simulink model "DrivetrainHevP2"  (R2018a)
settings: Solver=VariableStepAuto  StartTime=0.0  StopTime=inf  RelTol=1e-3  EnableMultiTasking=on
model workspace (MAT data in the model file):
  Aeff = 0.0314159265359
  Af = 2.46
  Bx = 10
  Cd = 0.25
  Cl = 0.1
  Cpm = 0.1
  Cx = 1.65
  Dx = 1
  Ex = 0.01
  FZMAX = 6570
  FZMIN = 0
  Fc = 500
  FsbF = [-700000 -7000 -700 0 700 7000 700000]
  FsbR = [-700000 -7000 -700 0 700 7000 700000]
  FskF = [-8928.57142857 -178.571428571 0 357.142857143 535.714285714 9285.71428571]
  FskR = [-5357.14285714 -107.142857143 0 214.285714286 321.428571429 5571.42857143]
  G = [0 1 2 3 4 5 6]
  G_o = 1
  Iyy = 3000
  Iyy_Whl = 0.8
  J = 0.01
  Jd = 0.025
  Jin = 0.05
  Jin_Cltch = 0.2
  Jin_Cltch2 = 0.01
  Jout = [0.01 0.01 0.01 0.01 0.01 0.01 0.01]
  Jout_Cltch = 0.01
  Jout_Cltch2 = 0.05
  Jw1 = 0.01
  Jw2 = 0.01
  K_c = 10000
  Lrel = 0.15
  Mass = 1623
  N = [1 4.212 2.637 1.8 1.386 1 0.772]
  NF = 2
  NR = 2
  Ndiff = 3.32
  Ndisk = 1
  Ndisks = 4
  Pabs = 101325
  Press = 7000000
  Re = 0.327
  Reff = 0.11
  Reff_LSD = 0.2
  Rm = 0.15
  T = 273
  UNLOADED_RADIUS = 0.336
  VXLOW = 2
  aMy = 0.01
  a_CG = 1.09
  alphaMy = 0
  b = Simulink.Parameter
  b.Value = 100
  b.DataType = 'auto'
  b.Dimensions = [1 1]
  b1 = 100
  b2 = 100
  bMy = 0
  b_CG = 1.7
  b_J = 0.001
  bd = 0.001
  betaMy = 1
  bin = 0.003
  bin_Cltch = 0.003
  bout = [0.003 0.003 0.003 0.003 0.003 0.003 0.003]
  bout_Cltch = 0.003
  br = 0.001
  bw1 = 0.001
  bw2 = 0.001
  cMy = 0
  disk_abore = 0.05
  domega_o = 0
  dw = [0 10 20 40 60 80 100]
  dzdotsF = [-10 -1 -0.1 0 0.1 1 10]
  dzdotsR = [-10 -1 -0.1 0 0.1 1 10]
  dzsF = [-0.005 -0.0001 0 0.2 0.2001 0.2051]
  dzsR = [-0.005 -0.0001 0 0.2 0.2001 0.2051]
  eta = [0.95 0.95 0.95 0.95 0.95 0.95 0.95]
  g = 9.81
  h = 0.5
  k = Simulink.Parameter
  k.Value = 5000
  k.DataType = 'auto'
  k.Dimensions = [1 1]
  k1 = 50000
  k2 = 50000
  kappamax = 1.5
  lam_x = 1
  mu_kinetic = 0.35
  mu_static = 0.45
  muc = [0.16 0.13 0.115 0.11 0.105 0.1025 0.10125]
  muk = 0.4
  mus = 0.45
  num_pads = 2
  omega1_c = 3000
  omega2_c = 3000
  omega_c = Simulink.Parameter
  omega_c.Value = 100
  omega_c.DataType = 'auto'
  omega_c.Dimensions = [1 1]
  omega_o_J = 0
  omegain_o = 0
  omegao = 0
  omegaout_o = 0
  omegaw1o = 0
  omegaw2o = 0
  press = 234400
  q_o = 0
  tauC = 0.1
  tauC_1 = 0.01
  tauC_LSD = 0.01
  tau_s = 0.1
  tc = 0.01
  theta_o = 0
  theta_o_Veh = 0
  ts = 0.01
  win_o = 0
  wout_o = 0
  x_o = 0
  xdot_o = 0
  z_o = -0.35
  zdot_o = 0
libraries: autolibsharedcoupling x8, autolibshared x7, autolibshareddiff x4, autolibtransamt x1, autolibcoupling x1
(part 1 of 4)
settings Model: ModifiedByFormat=The MathWorks, Inc.  PauseTimes=10  Creator=The MathWorks, Inc.  LastModifiedBy=The MathWorks, Inc.
settings SolverCC: AutoInsertRateTranBlk=on  DecoupledContinuousIntegration=on
settings DataIOCC: DSMLogging=off
settings ModelReferenceCC: PropagateSignalLabelsOutOfModel=off
settings CodeAppCC: StateflowObjectComments=on
settings GRTTargetCC: TargetLangStandard=C89/C90 (ANSI)
settings ConfigComp: CovMetricSettings=dsw  CovHtmlReporting=on  CovSaveCumulativeToWorkspaceVar=on  CovSaveSingleToWorkspaceVar=on  CovShowResultsExplorer=off  CovExternalEMLEnable=off
settings SimscapeCC: SimscapeNormalizeSystem=off

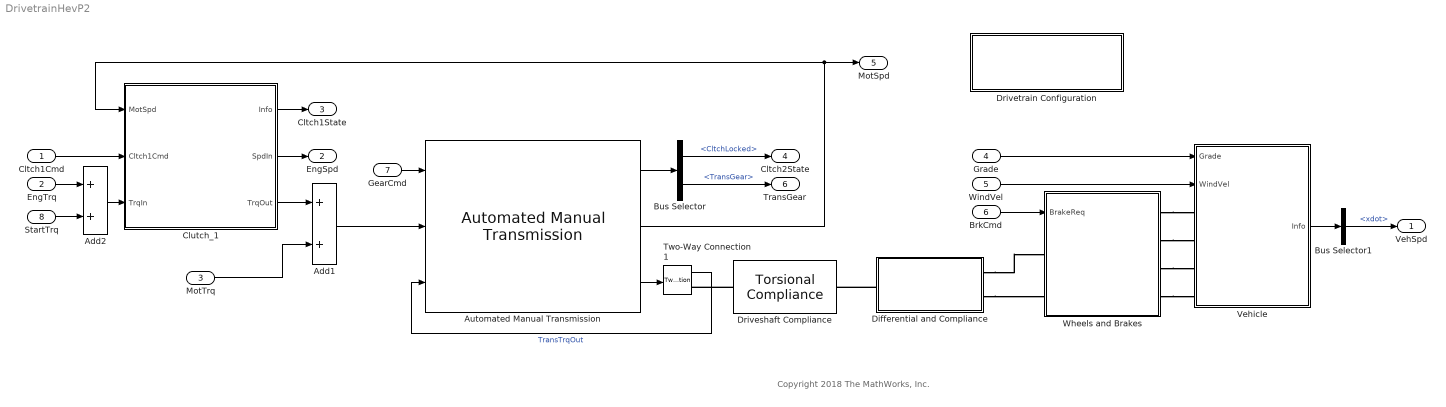
== system DrivetrainHevP2 ==
  note: Copyright 2018 The MathWorks, Inc.
  Cltch1Cmd : Inport
  EngTrq : Inport  Port=2
  MotTrq : Inport  Port=3
  Grade : Inport  Port=4
  WindVel : Inport  Port=5
  BrkCmd : Inport  Port=6
  GearCmd : Inport  Port=7
  StartTrq : Inport  Port=8
  Add1 : Sum
  Add2 : Sum
  Automated Manual Transmission : autolibtransamt/Automated Manual Transmission  VariantControl=0  cntrlType=Ideal integrated controller  TransEffModelPopup=Gear only  Jin=Jin  bin=bin  omegain_o=omegain_o  G=G  Trq_bpts=[25, 50, 75, 100, 150, 200, 250]  omega_bpts=[52.4 78.5 105 131 157 183 209 262 314 419 524]  Temp_bpts=[313 358]  N=N  Jout=Jout  bout=bout  eta=eta  eta_tbl=reshape([0.53 0.71 0.77 0.79 0.82 0.82 0.82 0.5 0.7 0.77 0.79 0.82 0.82 0.82 0.54 0.72 0.78 0.81 0.83 0.82 0.82 0.56 0.73 0.79 0.81 0.84 0.82 0.82 0.58 0.74 0.79 0.82 0.84 0.82 0.82 0.57 0.74 0.79 0.82 0.84 0.82 0.82 0.58 0.74 0.79 0.82 0.84 0.82 0.82 0.58 0.74 0.79 0.82 0.84 0.82 0.82 0.57 0.74 0.8 0.82 0.85 0.82 0.82 0.55 0.73 0.78 0.81 0.84 0.82 0.82 0.51 0.71 0.77 0.81 0.84 0.82 0.82 0.53 0.71 0.77 0.79 0.82 0.82 0.82 0.5 0.7 0.77 0.79 0.82 0.82 0.82 0.54 0.72 0.78 0.81 0.83 0.82 0.82 0.56 0.73 0.79 0.81 0.84 0.82 0.82 0.58 0.74 0.79 0.82 0.84 0.82 0.82 0.57 0.74 0.79 0.82 0.84 0.82 0.82 0.58 0.74 0.79 0.82 0.84 0.82 0.82 0.58 0.74 0.79 0.82 0.84 0.82 0.82 0.57 0.74 0.8 0.82 0.85 0.82 0.82 0.55 0.73 0.78 0.81 0.84 0.82 0.82 0.51 0.71 0.77 0.81 0.84 0.82 0.82 0.53 0.71 0.77 0.79 0.82 0.82 0.82 0.5 0.7 0.77 0.79 0.82 0.82 0.82 0.54 0.72 0.78 0.81 0.83 0.82 0.82 0.56 0.73 0.79 0.81 0.84 0.82 0.82 0.58 0.74 0.79 0.82 0.84 0.82 0.82 0.57 0.74 0.79 0.82 0.84 0.82 0.82 0.58 0.74 0.79 0.82 0.84 0.82 0.82 0.58 0.74 0.79 0.82 0.84 0.82 0.82 0.57 0.74 0.8 0.82 0.85 0.82 0.82 0.55 0.73 0.78 0.81 0.84 0.82 0.82 0.51 0.71 0.77 0.81 0.84 0.82 0.82 0.7 0.79 0.82 0.83 0.84 0.84 0.84 0.63 0.76 0.8 0.82 0.83 0.84 0.84 0.58 0.74 0.79 0.81 0.83 0.84 0.84 0.58 0.74 0.79 0.81 0.83 0.84 0.84 0.58 0.74 0.79 0.81 0.84 0.84 0.84 0.57 0.73 0.78 0.81 0.84 0.85 0.84 0.57 0.73 0.79 0.81 0.84 0.85 0.84 0.56 0.73 0.78 0.81 0.83 0.85 0.84 0.55 0.73 0.78 0.81 0.84 0.85 0.84 0.52 0.71 0.77 0.8 0.83 0.85 0.84 0.48 0.69 0.76 0.79 0.83 0.84 0.84 0.64 0.76 0.8 0.81 0.83 0.84 0.84 0.56 0.73 0.78 0.8 0.83 0.84 0.84 0.54 0.71 0.77 0.8 0.82 0.84 0.84 0.53 0.71 0.77 0.8 0.83 0.84 0.84 0.51 0.71 0.77 0.8 0.83 0.84 0.85 0.52 0.7 0.77 0.8 0.83 0.84 0.85 0.51 0.71 0.76 0.79 0.83 0.84 0.85 0.5 0.69 0.76 0.79 0.82 0.84 0.85 0.45 0.68 0.75 0.78 0.82 0.84 0.85 0.43 0.67 0.74 0.78 0.81 0.83 0.84 0.38 0.63 0.71 0.75 0.8 0.82 0.83 0.65 0.79 0.84 0.85 0.88 0.89 0.89 0.56 0.75 0.81 0.83 0.86 0.88 0.89 0.52 0.72 0.79 0.83 0.86 0.88 0.88 0.51 0.72 0.79 0.83 0.86 0.88 0.89 0.49 0.71 0.78 0.82 0.86 0.88 0.89 0.47 0.7 0.78 0.82 0.86 0.87 0.88 0.45 0.69 0.77 0.81 0.85 0.87 0.88 0.4 0.67 0.75 0.8 0.84 0.86 0.88 0.3 0.64 0.73 0.78 0.83 0.86 0.87 0.17 0.55 0.67 0.73 0.8 0.83 0.85 0.089 0.45 0.61 0.69 0.77 0.81 0.83 0.61 0.75 0.82 0.84 0.87 0.87 0.88 0.54 0.73 0.8 0.82 0.86 0.87 0.88 0.51 0.71 0.79 0.82 0.86 0.87 0.88 0.52 0.72 0.79 0.82 0.86 0.87 0.89 0.52 0.72 0.8 0.83 0.86 0.88 0.89 0.53 0.72 0.79 0.82 0.86 0.87 0.89 0.5 0.7 0.78 0.82 0.86 0.88 0.88 0.46 0.69 0.77 0.81 0.85 0.87 0.88 0.4 0.67 0.75 0.8 0.83 0.86 0.88 0.33 0.64 0.73 0.78 0.83 0.85 0.87 0.33 0.64 0.73 0.78 0.83 0.85 0.87 0.78 0.85 0.87 0.88 0.89 0.89 0.89 0.73 0.83 0.86 0.88 0.89 0.89 0.89 0.72 0.83 0.86 0.88 0.89 0.89 0.89 0.72 0.83 0.87 0.89 0.9 0.89 0.89 0.72 0.83 0.87 0.88 0.9 0.89 0.89 0.71 0.83 0.87 0.88 0.9 0.89 0.89 0.71 0.83 0.86 0.88 0.9 0.89 0.89 0.7 0.82 0.86 0.88 0.9 0.89 0.89 0.69 0.82 0.86 0.88 0.9 0.89 0.89 0.67 0.81 0.86 0.88 0.9 0.89 0.89 0.63 0.79 0.85 0.87 0.89 0.89 0.89 0.78 0.85 0.87 0.88 0.89 0.89 0.89 0.73 0.83 0.86 0.88 0.89 0.89 0.89 0.72 0.83 0.86 0.88 0.89 0.89 0.89 0.72 0.83 0.87 0.89 0.9 0.89 0.89 0.72 0.83 0.87 0.88 0.9 0.89 0.89 0.71 0.83 0.87 0.88 0.9 0.89 0.89 0.71 0.83 0.86 0.88 0.9 0.89 0.89 0.7 0.82 0.86 0.88 0.9 0.89 0.89 0.69 0.82 0.86 0.88 0.9 0.89 0.89 0.67 0.81 0.86 0.88 0.9 0.89 0.89 0.63 0.79 0.85 0.87 0.89 0.89 0.89 0.78 0.85 0.87 0.88 0.89 0.89 0.89 0.73 0.83 0.86 0.88 0.89 0.89 0.89 0.72 0.83 0.86 0.88 0.89 0.89 0.89 0.72 0.83 0.87 0.89 0.9 0.89 0.89 0.72 0.83 0.87 0.88 0.9 0.89 0.89 0.71 0.83 0.87 0.88 0.9 0.89 0.89 0.71 0.83 0.86 0.88 0.9 0.89 0.89 0.7 0.82 0.86 0.88 0.9 0.89 0.89 0.69 0.82 0.86 0.88 0.9 0.89 0.89 0.67 0.81 0.86 0.88 0.9 0.89 0.89 0.63 0.79 0.85 0.87 0.89 0.89 0.89 0.82 0.87 0.88 0.89 0.89 0.89 0.89 0.81 0.87 0.89 0.89 0.9 0.9 0.89 0.76 0.85 0.87 0.89 0.9 0.89 0.89 0.72 0.83 0.86 0.88 0.89 0.89 0.89 0.72 0.83 0.86 0.88 0.89 0.9 0.89 0.71 0.82 0.86 0.88 0.89 0.9 ...(+1314 chars))  omegaout_o=omegaout_o  G_o=G_o  tauc=tauC  ts=ts  tc=tc  R=Reff  K_c=K_c  mus=mus  muk=muk  ClutchLocked=off  SynchLocked=off  maxAbsSpd=5e3
      settings: SourceProductName=Powertrain Blockset  SourceProductBaseCode=PW
  Bus Selector : BusSelector  OutputSignals=Cltch.CltchLocked,Trans.TransGear
  Bus Selector1 : BusSelector  OutputSignals=BdyFrm.Cg.Vel.xdot
  Clutch_1 : Subsystem
  Differential and Compliance : Subsystem  Variant=on  OverrideUsingVariant=0
  Driveshaft Compliance : autolibsharedcoupling/Torsional Compliance  port_config=Two-way connection  k=k  b=b  theta_o=theta_o  domega_o=domega_o  omega_c=omega_c  blkID=0  aMode=1
      settings: SourceProductName=Powertrain Blockset
  Drivetrain Configuration : Subsystem  mask(Drivetrain Configuration){drivetrainMode=Front Wheel Drive}
      mask prompts: drivetrainMode "Drivetrain Mode"
      mask help: Use this block to configure the dirvetrain mode.
      settings: AttributesFormatString=Active Mode: %<drivetrainMode>
      mask TypeOptions drivetrainMode: Front Wheel Drive | Rear Wheel Drive | All Wheel Drive
      mask Callback drivetrainMode:
      | switch get_param(gcb,'drivetrainMode')
      |     case 'Front Wheel Drive'
      |         set_param([bdroot '/Wheels and Brakes'],'OverrideUsingVariant','0')
      |         set_param([bdroot '/Differential and Compliance'],'OverrideUsingVariant','0')
      |     case 'Rear Wheel Drive'
      |         set_param([bdroot '/Wheels and Brakes'],'OverrideUsingVariant','1')
      |         set_param([bdroot '/Differential and Compliance'],'OverrideUsingVariant','1')
      |     case 'All Wheel Drive'
      |         set_param([bdroot '/Wheels and Brakes'],'OverrideUsingVariant','2')
      |         set_param([bdroot '/Differential and Compliance'],'OverrideUsingVariant','2')
      |     otherwise
      |         set_param([bdroot '/Wheels and Brakes'],'OverrideUsingVariant','0')
      |         set_param([bdroot '/Differential and Compliance'],'OverrideUsingVariant','0')
      | end
      mask Display: disp('Double click to configure drivetrain')
  Two-Way Connection1 : TwoWayConnection
  Vehicle : Subsystem
  Wheels and Brakes : Subsystem  Variant=on  OverrideUsingVariant=0
  VehSpd : Outport
  EngSpd : Outport  Port=2  BusOutputAsStruct=on
  Cltch1State : Outport  Port=3  BusOutputAsStruct=on
  Cltch2State : Outport  Port=4  BusOutputAsStruct=on
  MotSpd : Outport  Port=5  BusOutputAsStruct=on
  TransGear : Outport  Port=6  BusOutputAsStruct=on
  wires:
  BrkCmd/1 -> Wheels and Brakes/1(BrakeReq)
  Automated Manual Transmission/3 -> Two-Way Connection1/1
  GearCmd/1 -> Automated Manual Transmission/1
  Two-Way Connection1/1 -> Automated Manual Transmission/3  "TransTrqOut"
  Grade/1 -> Vehicle/1(Grade)
  WindVel/1 -> Vehicle/2(WindVel)
  MotTrq/1 -> Add1/2
  Cltch1Cmd/1 -> Clutch_1/2(Cltch1Cmd)
  EngTrq/1 -> Add2/1
  Clutch_1/2(SpdIn) -> EngSpd/1
  Clutch_1/3(TrqOut) -> Add1/1
  Vehicle/1(Info) -> Bus Selector1/1
  Bus Selector1/1 -> VehSpd/1  "<xdot>"
  StartTrq/1 -> Add2/2
  Add2/1 -> Clutch_1/3(TrqIn)
  Automated Manual Transmission/2 -> Clutch_1/1(MotSpd), MotSpd/1
  Clutch_1/1(Info) -> Cltch1State/1
  Automated Manual Transmission/1 -> Bus Selector/1
  Bus Selector/1 -> Cltch2State/1  "<CltchLocked>"
  Add1/1 -> Automated Manual Transmission/2
  Bus Selector/2 -> TransGear/1  "<TransGear>"
  connections:
  Wheels and Brakes/RConn2 -- Vehicle/LConn2
  Wheels and Brakes/RConn1 -- Vehicle/LConn1
  Wheels and Brakes/RConn4 -- Vehicle/LConn4
  Wheels and Brakes/RConn3 -- Vehicle/LConn3
  Differential and Compliance/LConn1 -- Driveshaft Compliance/RConn1
  Driveshaft Compliance/LConn1 -- Two-Way Connection1/RConn1
  Differential and Compliance/RConn1 -- Wheels and Brakes/LConn1
  Differential and Compliance/RConn2 -- Wheels and Brakes/LConn2

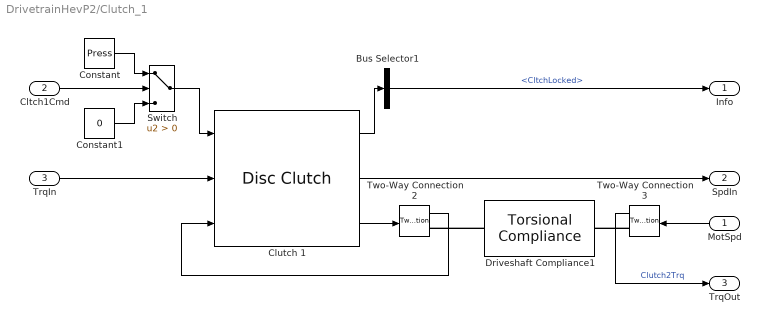
== system DrivetrainHevP2/Clutch_1 ==
  MotSpd : Inport
  Cltch1Cmd : Inport  Port=2
  TrqIn : Inport  Port=3
  Bus Selector1 : BusSelector  OutputSignals=Cltch.CltchLocked
  Clutch 1 : autolibcoupling/Disc Clutch  port_config=Simulink  Reff=Reff  Ndisk=Ndisk  Aeff=Aeff  Jin=Jin_Cltch  Jout=Jout_Cltch  muk=muk  mus=mus  bin=bin_Cltch  bout=bout_Cltch  win_o=win_o  wout_o=wout_o  tauC=tauC_1  InitiallyLocked=off  maxAbsSpd=3000  blkID=1
      settings: SourceProductName=Powertrain Blockset  SourceProductBaseCode=PW
  Constant : Constant  Value=Press
  Constant1 : Constant  Value=0
  Driveshaft Compliance1 : autolibsharedcoupling/Torsional Compliance  port_config=Two-way connection  k=k  b=b  theta_o=theta_o  domega_o=domega_o  omega_c=omega_c  blkID=0  aMode=1
      settings: SourceProductName=Powertrain Blockset
  Switch : Switch  Criteria=u2 > Threshold
  Two-Way Connection2 : TwoWayConnection
  Two-Way Connection3 : TwoWayConnection
  Info : Outport
  SpdIn : Outport  Port=2
  TrqOut : Outport  Port=3
  wires:
  MotSpd/1 -> Two-Way Connection3/1
  Two-Way Connection3/1 -> TrqOut/1  "Clutch2Trq"
  Constant/1 -> Switch/1
  Cltch1Cmd/1 -> Switch/2
  Constant1/1 -> Switch/3
  Two-Way Connection2/1 -> Clutch 1/3
  Clutch 1/3 -> Two-Way Connection2/1
  Clutch 1/1 -> Bus Selector1/1
  Clutch 1/2 -> SpdIn/1
  Bus Selector1/1 -> Info/1  "<CltchLocked>"
  TrqIn/1 -> Clutch 1/2
  Switch/1 -> Clutch 1/1
  connections:
  Two-Way Connection3/RConn1 -- Driveshaft Compliance1/RConn1
  Driveshaft Compliance1/LConn1 -- Two-Way Connection2/RConn1

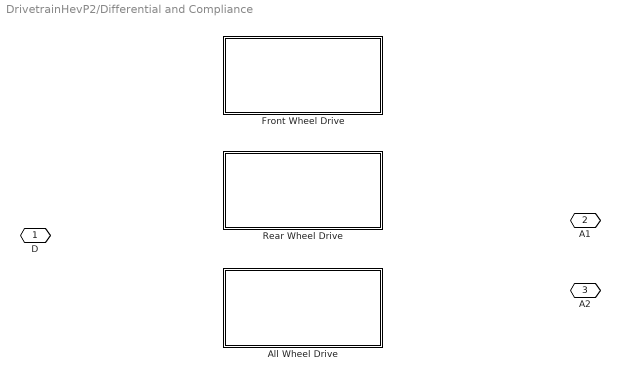
== system DrivetrainHevP2/Differential and Compliance ==
  All Wheel Drive : Subsystem  VariantControl=2
  Front Wheel Drive : Subsystem  VariantControl=0
  Rear Wheel Drive : Subsystem  VariantControl=1
  D : PMIOPort  Side=Left
  A1 : PMIOPort  Port=2  Side=Right
  A2 : PMIOPort  Port=3  Side=Right

== system DrivetrainHevP2/Drivetrain Configuration ==

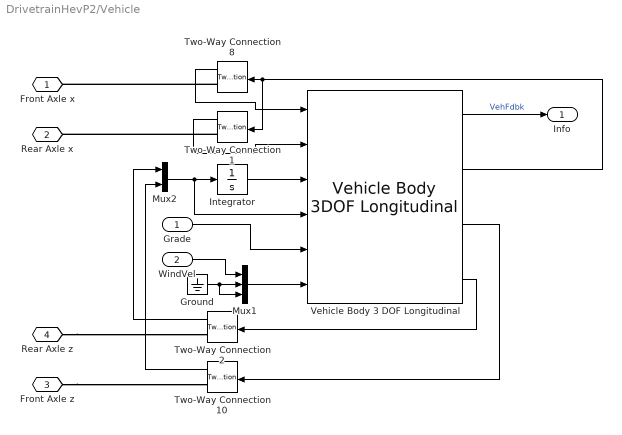
== system DrivetrainHevP2/Vehicle ==
  Grade : Inport
  WindVel : Inport  Port=2
  Ground : Ground
  Integrator : Integrator
  Mux1 : Mux  Inputs=3
  Mux2 : Mux  Inputs=2
  Two-Way Connection{1..2,8,10} (4 alike) : TwoWayConnection
  Vehicle Body 3 DOF Longitudinal : autolibshared/Vehicle Body 3DOF Longitudinal  VariantControl=SL  groundType=Axle displacement, velocity  aMode=aMode  NF=NF  NR=NR  m=Mass  a=a_CG  b=b_CG  h=h  Cd=Cd  Af=Af  x_o=x_o  xdot_o=xdot_o  Cl=Cl  z_o=z_o  zdot_o=zdot_o  Iyy=Iyy  Cpm=Cpm  theta_o=theta_o_Veh  q_o=q_o  FskF=FskF  dzsF=dzsF  FsbF=FsbF  dzdotsF=dzdotsF  FskR=FskR  dzsR=dzsR  FsbR=FsbR  dzdotsR=dzdotsR  Pabs=Pabs  T=T  g=g  blkID=0
      settings: SourceProductName=Powertrain Blockset  SourceProductBaseCode=PW
  Front Axle x : PMIOPort  Side=Left
  Rear Axle x : PMIOPort  Port=2  Side=Left
  Front Axle z : PMIOPort  Port=3  Side=Left
  Rear Axle z : PMIOPort  Port=4  Side=Left
  Info : Outport
  wires:
  Vehicle Body 3 DOF Longitudinal/3 -> Two-Way Connection10/1
  Vehicle Body 3 DOF Longitudinal/2 -> Two-Way Connection1/1, Two-Way Connection8/1
  Two-Way Connection8/1 -> Vehicle Body 3 DOF Longitudinal/1
  Vehicle Body 3 DOF Longitudinal/1 -> Info/1  "VehFdbk"
  Ground/1 -> Mux1/2, Mux1/3
  Mux1/1 -> Vehicle Body 3 DOF Longitudinal/6
  Two-Way Connection1/1 -> Vehicle Body 3 DOF Longitudinal/2
  Vehicle Body 3 DOF Longitudinal/4 -> Two-Way Connection2/1
  Two-Way Connection2/1 -> Mux2/1
  Two-Way Connection10/1 -> Mux2/2
  Mux2/1 -> Integrator/1, Vehicle Body 3 DOF Longitudinal/4
  Integrator/1 -> Vehicle Body 3 DOF Longitudinal/3
  Grade/1 -> Vehicle Body 3 DOF Longitudinal/5
  WindVel/1 -> Mux1/1
  connections:
  Two-Way Connection8/RConn1 -- Front Axle x/RConn1
  Front Axle z/RConn1 -- Two-Way Connection10/RConn1
  Two-Way Connection1/RConn1 -- Rear Axle x/RConn1
  Rear Axle z/RConn1 -- Two-Way Connection2/RConn1

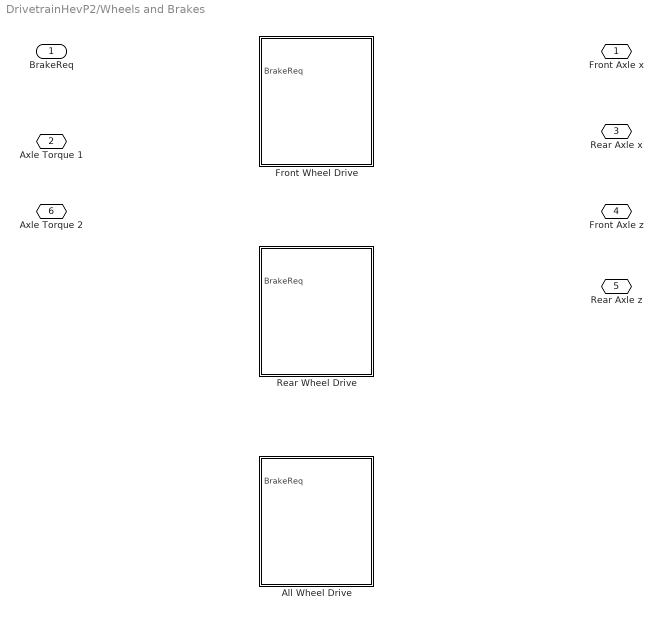
== system DrivetrainHevP2/Wheels and Brakes ==
  BrakeReq : Inport
  All Wheel Drive : Subsystem  VariantControl=2
  Front Wheel Drive : Subsystem  VariantControl=0
  Rear Wheel Drive : Subsystem  VariantControl=1
  Front Axle x : PMIOPort  Side=Right
  Axle Torque 1 : PMIOPort  Port=2  Side=Left
  Rear Axle x : PMIOPort  Port=3  Side=Right
  Front Axle z : PMIOPort  Port=4  Side=Right
  Rear Axle z : PMIOPort  Port=5  Side=Right
  Axle Torque 2 : PMIOPort  Port=6  Side=Left

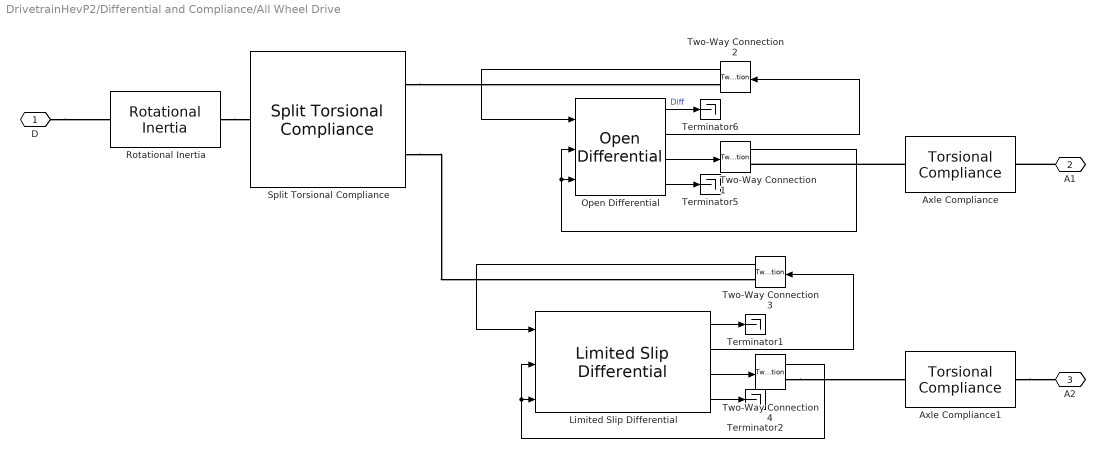
== system DrivetrainHevP2/Differential and Compliance/All Wheel Drive ==
  Axle Compliance : autolibsharedcoupling/Torsional Compliance  port_config=Two-way connection  k=k  b=b  theta_o=theta_o  domega_o=domega_o  omega_c=omega_c  blkID=0
      settings: SourceProductName=Powertrain Blockset
  Axle Compliance1 : autolibsharedcoupling/Torsional Compliance  port_config=Two-way connection  k=k  b=b  theta_o=theta_o  domega_o=domega_o  omega_c=omega_c  blkID=0
      settings: SourceProductName=Powertrain Blockset
  Limited Slip Differential : autolibshareddiff/Limited Slip Differential  shaftSwitchMask=To the left of center-line  Ndiff=Ndiff  Jd=Jd  bd=bd  Jw1=Jw1  bw1=bw1  Jw2=Jw2  bw2=bw2  omegaw1o=omegaw1o  omegaw2o=omegaw2o  couplingType=Pre-loaded ideal clutch  Ndisks=Ndisks  Reff=Reff_LSD  Fc=Fc  muc=muc  dw=dw  IdealInterpMethod=Linear  IdealExtrapMethod=Linear  Tdw=[-100, -90, -50, -5, 0, 5, 50, 90, 100]  dwT=[-200, -175, -100, - 50, 0, 50, 100, 175, 200]  TdwInterpMethod=Linear  TdwExtrapMethod=Linear  TTin=[-200 -175 -100 - 50 0 50 100 175 200]  Tin=[-200 -175 -100 - 50 0 50 100 175 200]  TTinInterpMethod=Linear  TTinExtrapMethod=Linear  tauC=tauC_LSD  maxAbsSpd=5e3
      settings: SourceProductName=Powertrain Blockset  SourceProductBaseCode=PW
  Open Differential : autolibshareddiff/Open Differential  shaftSwitchMask=To the left of center-line  Ndiff=Ndiff  Jd=Jd  bd=bd  Jw1=Jw1  bw1=bw1  Jw2=Jw2  bw2=bw2  omegaw1o=omegaw1o  omegaw2o=omegaw2o  maxAbsSpd=5e3
      settings: SourceProductName=Powertrain Blockset
  Rotational Inertia : autolibsharedcoupling/Rotational Inertia  port_config=Two-way connection  J=J  b=b_J  omega_o=omega_o_J  externJ=off  blkID=0
      settings: SourceProductName=Powertrain Blockset  SourceProductBaseCode=PW
  Split Torsional Compliance : autolibsharedcoupling/Split Torsional Compliance  port_config=Two-way connection  cplrMode=Shaft split  k1=k1  b1=b1  omega1_c=omega1_c  theta1_o=0  domega1_o=0  k2=k2  b2=b2  omega2_c=omega2_c  theta2_o=0  domega2_o=0  blkID=0
      settings: SourceProductName=Powertrain Blockset  SourceProductBaseCode=PW
  Terminator{1..2,5..6} (4 alike) : Terminator
  Two-Way Connection{1..4} (4 alike) : TwoWayConnection
  D : PMIOPort  Side=Left
  A1 : PMIOPort  Port=2  Side=Right
  A2 : PMIOPort  Port=3  Side=Right
  wires:
  Open Differential/1 -> Terminator6/1  "Diff"
  Two-Way Connection2/1 -> Open Differential/1
  Two-Way Connection1/1 -> Open Differential/2, Open Differential/3
  Open Differential/3 -> Two-Way Connection1/1
  Open Differential/4 -> Terminator5/1
  Open Differential/2 -> Two-Way Connection2/1
  Two-Way Connection3/1 -> Limited Slip Differential/1
  Limited Slip Differential/1 -> Terminator1/1
  Limited Slip Differential/3 -> Two-Way Connection4/1
  Two-Way Connection4/1 -> Limited Slip Differential/3, Limited Slip Differential/2
  Limited Slip Differential/2 -> Two-Way Connection3/1
  Limited Slip Differential/4 -> Terminator2/1
  connections:
  D/RConn1 -- Rotational Inertia/LConn1
  Split Torsional Compliance/RConn1 -- Two-Way Connection2/RConn1
  Axle Compliance/LConn1 -- Two-Way Connection1/RConn1
  A1/RConn1 -- Axle Compliance/RConn1
  Split Torsional Compliance/RConn2 -- Two-Way Connection3/RConn1
  Axle Compliance1/RConn1 -- A2/RConn1
  Two-Way Connection4/RConn1 -- Axle Compliance1/LConn1
  Rotational Inertia/RConn1 -- Split Torsional Compliance/LConn1

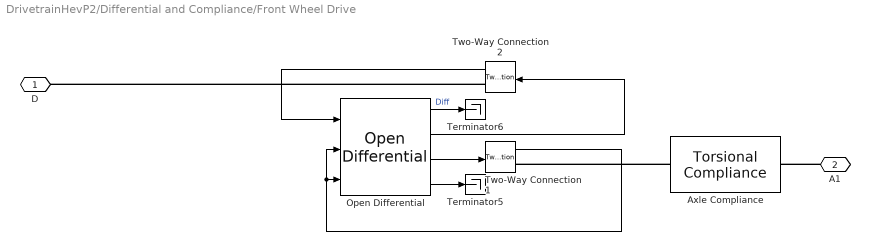
== system DrivetrainHevP2/Differential and Compliance/Front Wheel Drive ==
  Axle Compliance : autolibsharedcoupling/Torsional Compliance  port_config=Two-way connection  k=k  b=b  theta_o=theta_o  domega_o=domega_o  omega_c=omega_c  blkID=0  aMode=1
      settings: SourceProductName=Powertrain Blockset
  Open Differential : autolibshareddiff/Open Differential  shaftSwitchMask=To the left of center-line  Ndiff=Ndiff  Jd=Jd  bd=bd  Jw1=Jw1  bw1=bw1  Jw2=Jw2  bw2=bw2  omegaw1o=omegaw1o  omegaw2o=omegaw2o  maxAbsSpd=5e3  aMode=1
      settings: SourceProductName=Powertrain Blockset
  Terminator5 : Terminator
  Terminator6 : Terminator
  Two-Way Connection1 : TwoWayConnection
  Two-Way Connection2 : TwoWayConnection
  D : PMIOPort  Side=Left
  A1 : PMIOPort  Port=2  Side=Right
  wires:
  Open Differential/1 -> Terminator6/1  "Diff"
  Two-Way Connection2/1 -> Open Differential/1
  Two-Way Connection1/1 -> Open Differential/2, Open Differential/3
  Open Differential/3 -> Two-Way Connection1/1
  Open Differential/4 -> Terminator5/1
  Open Differential/2 -> Two-Way Connection2/1
  connections:
  A1/RConn1 -- Axle Compliance/RConn1
  Axle Compliance/LConn1 -- Two-Way Connection1/RConn1
  Two-Way Connection2/RConn1 -- D/RConn1

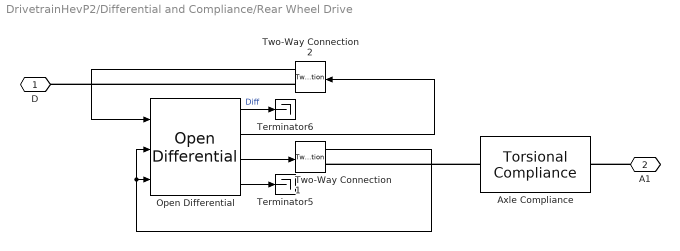
== system DrivetrainHevP2/Differential and Compliance/Rear Wheel Drive ==
  Axle Compliance : autolibsharedcoupling/Torsional Compliance  port_config=Two-way connection  k=k  b=b  theta_o=theta_o  domega_o=domega_o  omega_c=omega_c  blkID=0
      settings: SourceProductName=Powertrain Blockset
  Open Differential : autolibshareddiff/Open Differential  shaftSwitchMask=To the left of center-line  Ndiff=Ndiff  Jd=Jd  bd=bd  Jw1=Jw1  bw1=bw1  Jw2=Jw2  bw2=bw2  omegaw1o=omegaw1o  omegaw2o=omegaw2o  maxAbsSpd=5e3
      settings: SourceProductName=Powertrain Blockset
  Terminator5 : Terminator
  Terminator6 : Terminator
  Two-Way Connection1 : TwoWayConnection
  Two-Way Connection2 : TwoWayConnection
  D : PMIOPort  Side=Left
  A1 : PMIOPort  Port=2  Side=Right
  wires:
  Open Differential/1 -> Terminator6/1  "Diff"
  Two-Way Connection2/1 -> Open Differential/1
  Two-Way Connection1/1 -> Open Differential/2, Open Differential/3
  Open Differential/3 -> Two-Way Connection1/1
  Open Differential/4 -> Terminator5/1
  Open Differential/2 -> Two-Way Connection2/1
  connections:
  A1/RConn1 -- Axle Compliance/RConn1
  Axle Compliance/LConn1 -- Two-Way Connection1/RConn1
  Two-Way Connection2/RConn1 -- D/RConn1
